simulink model "Car"  (Simulink 7.4)
settings: Solver=ode45  StartTime=0.0  StopTime=28  MaxStep=0.2  MinStep=0.1  RelTol=1e-3
values from neighbouring files (symbols this model uses):
  g = 9.81    [parameters.m]
  J_w = 9.55    [parameters.m]
  m = 300    [parameters.m]
  R = 0.32    [parameters.m]
  r_k = 0.32    [parameters.m]
libraries: simulink x4
settings Model: Creator=Ozo  LastModifiedBy=Ozo

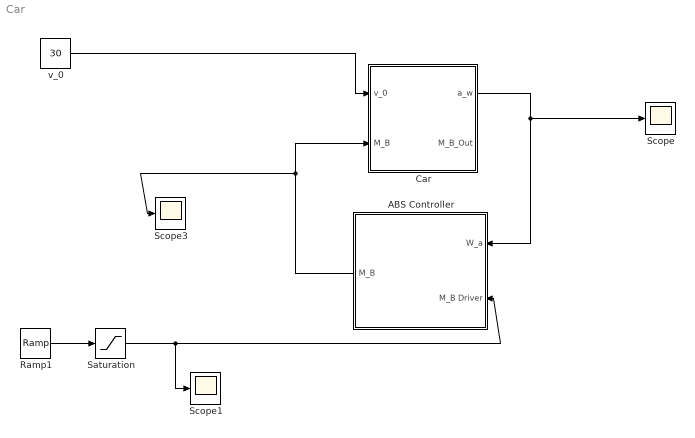
== system Car ==
  ABS Controller : Subsystem
  Car : Subsystem
  Ramp1 : simulink/Sources/Ramp  SystemSampleTime=-1  slope=50  start=0  X0=0
  Saturation : Saturate  UpperLimit=1200  OutDataType=fixdt(1, 16)  OutScaling=2^0
  Scope : Scope
      settings: TimeRange=5  YMin=-7
  Scope1 : Scope
  Scope3 : Scope
      settings: TimeRange=5  YMin=-60  YMax=10  SaveName=ScopeData11
  v_0 : Constant  Value=30  OutDataType=fixdt(1, 16)  OutScaling=2^0
  wires:
  Car/1(a_w) -> ABS Controller/1(W_a), Scope/1
  Ramp1/1 -> Saturation/1
  ABS Controller/1(M_B) -> Car/2(M_B), Scope3/1
  v_0/1 -> Car/1(v_0)
  Saturation/1 -> Scope1/1, ABS Controller/2(M_B Driver)

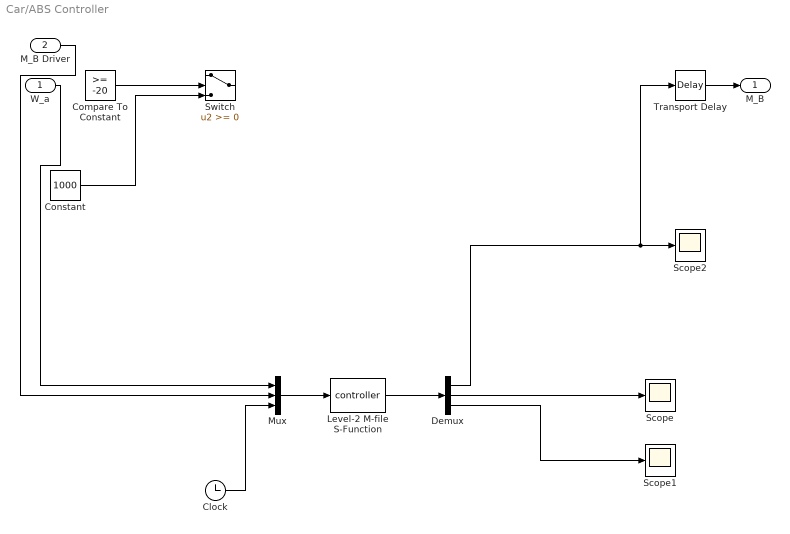
== system Car/ABS Controller ==
  W_a : Inport  OutDataType=fixdt(1, 16)  OutScaling=2^0
  M_B Driver : Inport  Port=2  OutDataType=fixdt(1, 16)  OutScaling=2^0
  Clock : Clock
      settings: Decimation=10
  Compare To Constant : simulink/Logic and Bit Operations/Compare To Constant  SystemSampleTime=-1  relop=>=  const=-20  LogicOutDataTypeMode=boolean
  Constant : Constant  Value=1000  OutDataType=fixdt(1, 16)  OutScaling=2^0
  Demux : Demux  Outputs=3
  Level-2 M-file S-Function : M-S-Function  FunctionName=controller
  Mux : Mux  Inputs=3
  Scope : Scope
      settings: YMin=0  YMax=3  SaveName=ScopeData3
  Scope1 : Scope
      settings: SaveName=ScopeData4
  Scope2 : Scope
      settings: YMin=0  YMax=900  SaveName=ScopeData12
  Switch : Switch  OutDataType=fixdt(1, 16)  OutScaling=2^0
  Transport Delay : TransportDelay  DelayTime=0.3
  M_B : Outport  OutDataType=fixdt(1, 16)  OutScaling=2^0
  wires:
  Mux/1 -> Level-2 M-file S-Function/1
  Level-2 M-file S-Function/1 -> Demux/1
  Clock/1 -> Mux/3
  Constant/1 -> Switch/3
  Compare To Constant/1 -> Switch/2
  Demux/1 -> Scope2/1, Transport Delay/1
  W_a/1 -> Mux/1
  M_B Driver/1 -> Mux/2
  Demux/2 -> Scope/1
  Demux/3 -> Scope1/1
  Transport Delay/1 -> M_B/1

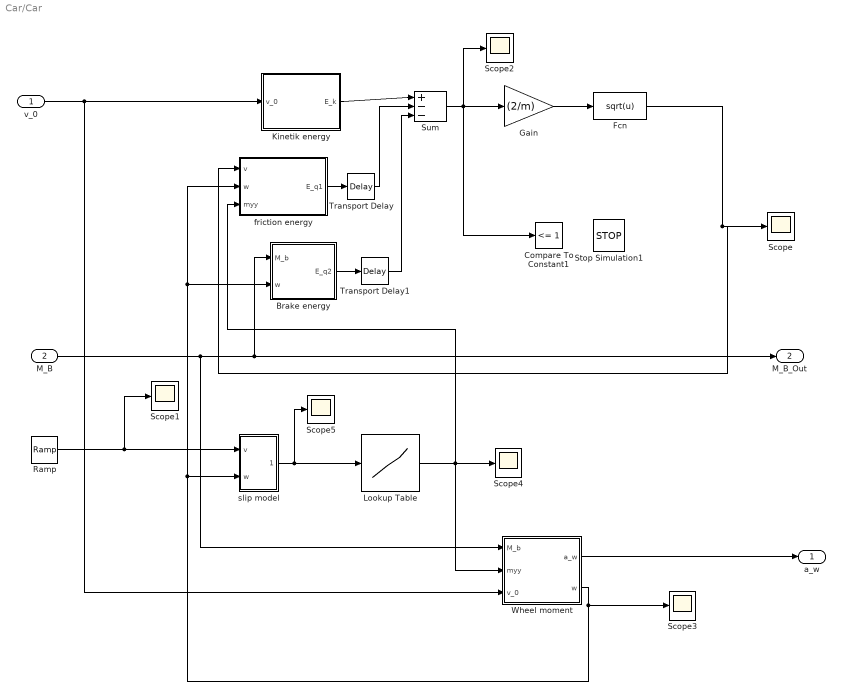
== system Car/Car ==
  v_0 : Inport  OutDataType=fixdt(1, 16)  OutScaling=2^0
  M_B : Inport  Port=2  OutDataType=fixdt(1, 16)  OutScaling=2^0
  Brake energy : Subsystem
  Compare To Constant1 : simulink/Logic and Bit Operations/Compare To Constant  SystemSampleTime=-1  relop=<=  const=1  LogicOutDataTypeMode=boolean
  Fcn : Fcn  Expr=sqrt(u)
  Gain : Gain  Gain=(2/m)  ParameterDataType=fixdt(1, 16)  ParameterScaling=2^0  OutDataType=fixdt(1, 16)  OutScaling=2^0
  Kinetik energy : Subsystem
  Lookup Table : Lookup  InputValues=[-1,-0.8,-0.6,-0.4,-0.2,0,0.2,0.4,0.6,0.8,1]  Table=[-0.6099092042625951,-0.629329299739067,-0.6550547536867305,-0.7240275800758169,-0.8015941559557649,0,0.8015941559557649,0.7240275800758169,0.6550547536867305,0.629329299739067,0.6099092042625951]  OutDataType=fixdt(1, 16)  OutScaling=2^0
  Ramp : simulink/Sources/Ramp  SystemSampleTime=-1  slope=-1  start=0.1  X0=30
  Scope{,1..5} (6 alike) : Scope
      Scope settings: SaveName=ScopeData2
      Scope1 settings: SaveName=ScopeData13
      Scope2 settings: SaveName=ScopeData5
      Scope3 settings: SaveName=ScopeData6
      Scope4 settings: SaveName=ScopeData7
      Scope5 settings: SaveName=ScopeData8
  Stop Simulation1 : Stop
  Sum : Sum  Inputs=|+--  OutDataType=fixdt(1, 16)  OutScaling=2^0
  Transport Delay : TransportDelay
  Transport Delay1 : TransportDelay
  Wheel moment : Subsystem
  friction energy : Subsystem
  slip model : Subsystem
  a_w : Outport  OutDataType=fixdt(1, 16)  OutScaling=2^0
  M_B_Out : Outport  Port=2  OutDataType=fixdt(1, 16)  OutScaling=2^0
  wires:
  Kinetik energy/1(E_k) -> Sum/1
  Sum/1 -> Scope2/1, Gain/1, Compare To Constant1/1
  Gain/1 -> Fcn/1
  Fcn/1 -> Scope/1, friction energy/1(v)
  v_0/1 -> Kinetik energy/1(v_0), Wheel moment/3(v_0)
  friction energy/1(E_q1) -> Transport Delay/1
  Brake energy/1(E_q2) -> Transport Delay1/1
  slip model/1(kappa) -> Scope5/1, Lookup Table/1
  Lookup Table/1 -> friction energy/3(myy), Scope4/1, Wheel moment/2(myy)
  Wheel moment/2(w) -> slip model/2(w), friction energy/2(w), Brake energy/2(w), Scope3/1
  Wheel moment/1(a_w) -> a_w/1
  M_B/1 -> Brake energy/1(M_b), M_B_Out/1, Wheel moment/1(M_b)
  Transport Delay/1 -> Sum/2
  Transport Delay1/1 -> Sum/3
  Ramp/1 -> Scope1/1, slip model/1(v)

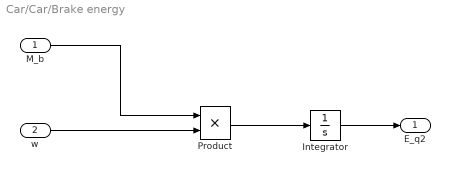
== system Car/Car/Brake energy ==
  M_b : Inport  OutDataType=fixdt(1, 16)  OutScaling=2^0
  w : Inport  Port=2  OutDataType=fixdt(1, 16)  OutScaling=2^0
  Integrator : Integrator
  Product : Product  OutDataType=fixdt(1, 16)  OutScaling=2^0  RndMeth=Zero
  E_q2 : Outport  OutDataType=fixdt(1, 16)  OutScaling=2^0
  wires:
  Product/1 -> Integrator/1
  M_b/1 -> Product/1
  w/1 -> Product/2
  Integrator/1 -> E_q2/1

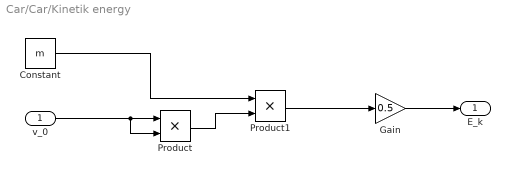
== system Car/Car/Kinetik energy ==
  v_0 : Inport  OutDataType=fixdt(1, 16)  OutScaling=2^0
  Constant : Constant  Value=m  OutDataType=fixdt(1, 16)  OutScaling=2^0
  Gain : Gain  Gain=0.5  ParameterDataType=fixdt(1, 16)  ParameterScaling=2^0  OutDataType=fixdt(1, 16)  OutScaling=2^0
  Product : Product  OutDataType=fixdt(1, 16)  OutScaling=2^0  RndMeth=Zero
  Product1 : Product  OutDataType=fixdt(1, 16)  OutScaling=2^0  RndMeth=Zero
  E_k : Outport  OutDataType=fixdt(1, 16)  OutScaling=2^0
  wires:
  v_0/1 -> Product/1, Product/2
  Product/1 -> Product1/2
  Constant/1 -> Product1/1
  Product1/1 -> Gain/1
  Gain/1 -> E_k/1

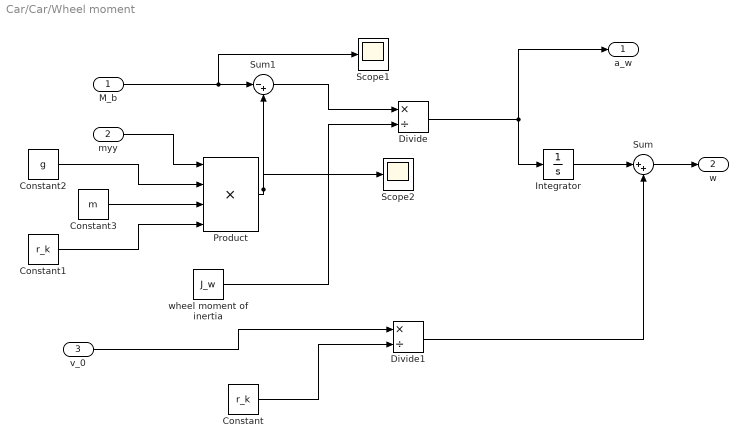
== system Car/Car/Wheel moment ==
  M_b : Inport  OutDataType=fixdt(1, 16)  OutScaling=2^0
  myy : Inport  Port=2  OutDataType=fixdt(1, 16)  OutScaling=2^0
  v_0 : Inport  Port=3  OutDataType=fixdt(1, 16)  OutScaling=2^0
  Constant : Constant  Value=r_k  OutDataType=fixdt(1, 16)  OutScaling=2^0
  Constant1 : Constant  Value=r_k  OutDataType=fixdt(1, 16)  OutScaling=2^0
  Constant2 : Constant  Value=g  OutDataType=fixdt(1, 16)  OutScaling=2^0
  Constant3 : Constant  Value=m  OutDataType=fixdt(1, 16)  OutScaling=2^0
  Divide : Product  Inputs=*/  OutDataType=fixdt(1, 16)  OutScaling=2^-10
  Divide1 : Product  Inputs=*/  OutDataType=fixdt(1, 16)  OutScaling=2^-10
  Integrator : Integrator
  Product : Product  Inputs=4  OutDataType=fixdt(1, 16)  OutScaling=2^0  RndMeth=Zero
  Scope1 : Scope
      settings: TimeRange=5  SaveName=ScopeData9
  Scope2 : Scope
      settings: SaveName=ScopeData10
  Sum : Sum  Inputs=|++  OutDataType=fixdt(1, 16)  OutScaling=2^0
  Sum1 : Sum  Inputs=|-+  OutDataType=fixdt(1, 16)  OutScaling=2^0
  wheel moment of inertia : Constant  Value=J_w  OutDataType=fixdt(1, 16)  OutScaling=2^0
  a_w : Outport  OutDataType=fixdt(1, 16)  OutScaling=2^0
  w : Outport  Port=2  OutDataType=fixdt(1, 16)  OutScaling=2^0
  wires:
  M_b/1 -> Sum1/1, Scope1/1
  myy/1 -> Product/1
  Constant2/1 -> Product/2
  Constant3/1 -> Product/3
  Constant1/1 -> Product/4
  Product/1 -> Sum1/2, Scope2/1
  Sum1/1 -> Divide/1
  wheel moment of inertia/1 -> Divide/2
  Integrator/1 -> Sum/1
  v_0/1 -> Divide1/1
  Constant/1 -> Divide1/2
  Divide1/1 -> Sum/2
  Sum/1 -> w/1
  Divide/1 -> Integrator/1, a_w/1

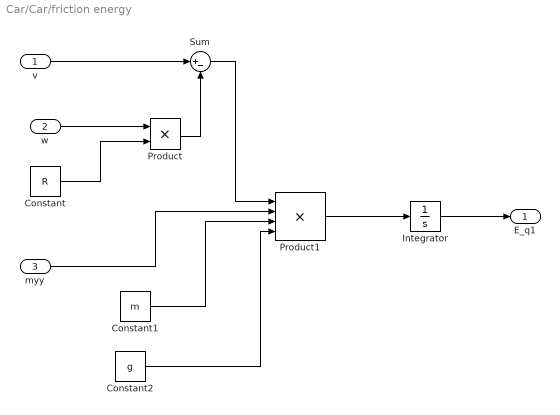
== system Car/Car/friction energy ==
  v : Inport  OutDataType=fixdt(1, 16)  OutScaling=2^0
  w : Inport  Port=2  OutDataType=fixdt(1, 16)  OutScaling=2^0
  myy : Inport  Port=3  OutDataType=fixdt(1, 16)  OutScaling=2^0
  Constant : Constant  Value=R  OutDataType=fixdt(1, 16)  OutScaling=2^0
  Constant1 : Constant  Value=m  OutDataType=fixdt(1, 16)  OutScaling=2^0
  Constant2 : Constant  Value=g  OutDataType=fixdt(1, 16)  OutScaling=2^0
  Integrator : Integrator
  Product : Product  OutDataType=fixdt(1, 16)  OutScaling=2^0  RndMeth=Zero
  Product1 : Product  Inputs=4  OutDataType=fixdt(1, 16)  OutScaling=2^0  RndMeth=Zero
  Sum : Sum  Inputs=|+-  OutDataType=fixdt(1, 16)  OutScaling=2^0
  E_q1 : Outport  OutDataType=fixdt(1, 16)  OutScaling=2^0
  wires:
  w/1 -> Product/1
  Constant/1 -> Product/2
  Product/1 -> Sum/2
  v/1 -> Sum/1
  Sum/1 -> Product1/1
  myy/1 -> Product1/2
  Constant1/1 -> Product1/3
  Constant2/1 -> Product1/4
  Product1/1 -> Integrator/1
  Integrator/1 -> E_q1/1

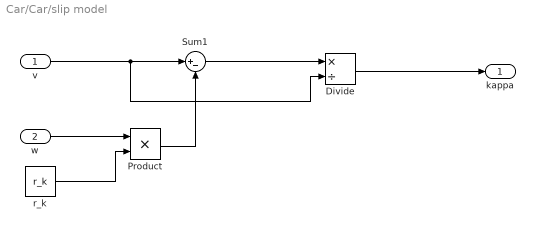
== system Car/Car/slip model ==
  v : Inport  OutDataType=fixdt(1, 16)  OutScaling=2^0
  w : Inport  Port=2  OutDataType=fixdt(1, 16)  OutScaling=2^0
  Divide : Product  Inputs=*/  OutDataType=fixdt(1, 16)  OutScaling=2^-10
  Product : Product  OutDataType=fixdt(1, 16)  OutScaling=2^0  RndMeth=Zero
  Sum1 : Sum  Inputs=|+-  OutDataType=fixdt(1, 16)  OutScaling=2^0
  r_k : Constant  Value=r_k  OutDataType=fixdt(1, 16)  OutScaling=2^0
  kappa : Outport  OutDataType=fixdt(1, 16)  OutScaling=2^0
  wires:
  r_k/1 -> Product/2
  w/1 -> Product/1
  v/1 -> Sum1/1, Divide/2
  Product/1 -> Sum1/2
  Sum1/1 -> Divide/1
  Divide/1 -> kappa/1
